simulink model "dynamicModel"  (R2016a)
settings: Solver=VariableStepAuto  StartTime=0.0  StopTime=10.0  RelTol=1e-3
settings Model: Creator=wfp  LastModifiedBy=wfp

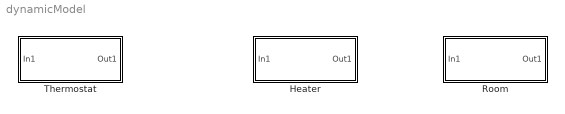
== system dynamicModel ==
  Heater : Subsystem
  Room : Subsystem
  Thermostat : Subsystem

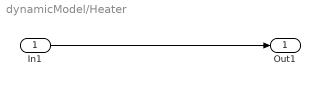
== system dynamicModel/Heater ==
  In1 : Inport
  Out1 : Outport
  wires:
  In1/1 -> Out1/1

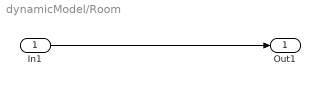
== system dynamicModel/Room ==
  In1 : Inport
  Out1 : Outport
  wires:
  In1/1 -> Out1/1

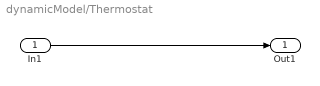
== system dynamicModel/Thermostat ==
  In1 : Inport
  Out1 : Outport
  wires:
  In1/1 -> Out1/1
